simulink model "SEBAS_mario"  (R2013b)
settings: Solver=FixedStepDiscrete  SolverMode=SingleTasking  StartTime=0.0  StopTime=inf  FixedStep=balancer_ts  RelTol=1e-3
undefined symbols (not defined in the file): a_d, a_r, balancerStates_Bus0, Batt, battery_gain, battery_offset, cmd_max, current_mode_status, current_task_operation_status, DiscIntNeverNeededParam, exec_period, Init_Bus0, K, k_f, k_i, k_phidot, k_thetadot, lightCalib, phi_des, R, STATE, TRACK_MODE_LIST, ts2, W
libraries: legonxtlib x29, simulink x19, simulink_extras x4
(part 5 of 5)

== stateflow chart SEBAS_mario/Main Controller/normal_operation_modes.line_tracking_mode ==
  state line_tracking_mode
    entry:
    desired_tail = single(2.0); %radian
    entry, during:
    PWM.tail = tail_controller(sensors.theta_T,desired_tail);
    exit:
    PWM.tail = single(0);
    state Waiting
      entry: debugFlag = uint16(400);
    state Track
      entry:
      BT_status_out = single(StatusID.NXT1_AT_STAGE);
      debugFlag = uint16(401);
      bias = single(0);
      FlagSteering = single(0);
      lineSide = single(1);
      desired_tail = single(0); %radian
      gyroTrick = single(0);
      minLight = lightCalib.flashingWhite;
      maxLight = lightCalib.flashingBlack;
      bias_WhiteSide = lightCalib.flashingWhite + 0.3*(lightCalib.flashingBlack - lightCalib.flashingWhite);
      bias_BlackSide = lightCalib.flashingBlack - 0.45*(lightCalib.flashingBlack - lightCalib.flashingWhite);
      state preProcess [parallel]
        during:
        on every(3, tick):
        [normalizedLight, filteredLight] = processLight(sensors.light, bias, minLight,maxLight);
        [AngleCount,EncoderReset,Angle, Distance] = analyzeEncoders(rawSensors);
        settings: executionOrder=1
      state manageRacePhases [parallel]
        settings: executionOrder=2
        state BeforeShortcut
          entry:
          PID = single([10 0 30 0 90]');
          FlagSteering = single(0);
          bias = single(0);
          state RocketStart1
            state Gyro [parallel]
              settings: executionOrder=1
              state trick
                entry: gyroTrick = single(20);
              state Normal
                entry: gyroTrick = single(0);
              (default) -> trick
              trick -> Normal : after(3*20*0.004,sec)
            state Speed [parallel]
              settings: executionOrder=2
              state slowdown
                entry: fwd = single(130)
                during:
                % fwd = fwd + single(0.005/3);
                fwd = fwd + single(1/2);
              state constantSpeed2
              (default) -> line_tracking_mode.Track.manageRacePhases.BeforeShortcut.RocketStart1.Speed.slowdown
              line_tracking_mode.Track.manageRacePhases.BeforeShortcut.RocketStart1.Speed.slowdown -> line_tracking_mode.Track.manageRacePhases.BeforeShortcut.RocketStart1.Speed.constantSpeed2 : [fwd >= 140]
          state GoUp
            entry:Speak;
            bias = bias_WhiteSide;
            state slowdown
              during:
              fwd = fwd - single(1/2);
            state constantSpeed1
            (default) -> line_tracking_mode.Track.manageRacePhases.BeforeShortcut.GoUp.slowdown
            line_tracking_mode.Track.manageRacePhases.BeforeShortcut.GoUp.slowdown -> line_tracking_mode.Track.manageRacePhases.BeforeShortcut.GoUp.constantSpeed1 : [fwd <= 120]
          state GoDown
            entry:Speak;
            bias = bias_BlackSide;
            state speedup
              during:
              % fwd = fwd + single(1/3)
              fwd = fwd + single(1/4)
            state constantSpeed1
            (default) -> speedup
            speedup -> line_tracking_mode.Track.manageRacePhases.BeforeShortcut.GoDown.constantSpeed1 : [fwd >= 130]
          state Curve
            entry:Speak;
            PID = single([20 0 30 0 100]');
            bias = bias_WhiteSide;
            state slowdown
              during:
              fwd = fwd - single(1/3)
            state constantSpeed2
            (default) -> line_tracking_mode.Track.manageRacePhases.BeforeShortcut.Curve.slowdown
            line_tracking_mode.Track.manageRacePhases.BeforeShortcut.Curve.slowdown -> line_tracking_mode.Track.manageRacePhases.BeforeShortcut.Curve.constantSpeed2 : [fwd <= 120]
          (default) -> RocketStart1
          RocketStart1 -> GoUp : [single(EncoderReset*(2*pi*4.1)/360) >= single(200)]
          GoUp -> GoDown : [single(EncoderReset*(2*pi*4.1)/360) >= single(270)]
          GoDown -> Curve : [single(EncoderReset*(2*pi*4.1)/360) >= single(410)]
        state Shortcut
          state Shortcut
            entry:
            Speak;
            PID = single([18 0 0 0 0]');
            FlagSteering = single(1);
            state slowdown
              during:
              fwd = fwd - single(2)
            state coast
            (default) -> line_tracking_mode.Track.manageRacePhases.Shortcut.Shortcut.slowdown
            line_tracking_mode.Track.manageRacePhases.Shortcut.Shortcut.slowdown -> line_tracking_mode.Track.manageRacePhases.Shortcut.Shortcut.coast : [fwd <= 60]
          state TurnTowardLine
            entry:
            Speak;
            PID = single([0 0 0 0 0]');
            FlagSteering = single(1);
          state skipFirstLine
            entry: Speak;
            EncoderTmp = EncoderReset;
          state SearchLine2
            state TurnLeft
              entry:
              Speak;
              PID = single([25 0 0 0 0]');
              FlagSteering = single(1);
              state slowdown
                during:
                fwd = fwd - single(2)
              state coast
              (default) -> line_tracking_mode.Track.manageRacePhases.Shortcut.SearchLine2.TurnLeft.slowdown
              line_tracking_mode.Track.manageRacePhases.Shortcut.SearchLine2.TurnLeft.slowdown -> line_tracking_mode.Track.manageRacePhases.Shortcut.SearchLine2.TurnLeft.coast : [fwd <= 20]
            state SlowlyApproachLine
              entry:
              Speak;
              fwd = single(20);
              PID = single([-2 0 0 0 0]');
              FlagSteering = single(1);
            (default) -> TurnLeft
            TurnLeft -> SlowlyApproachLine : [Angle >= single(245)]
          state SlowlyRestartLineTracking1
            entry: Speak;
            fwd = single(20);
            PID = single([30 0 25 0 100]');
            bias = single(0);
            FlagSteering = single(0);
          (default) -> line_tracking_mode.Track.manageRacePhases.Shortcut.Shortcut
          line_tracking_mode.Track.manageRacePhases.Shortcut.Shortcut -> TurnTowardLine : [Angle > single(205)]
          TurnTowardLine -> skipFirstLine : [filteredLight>single(0)]
          skipFirstLine -> SearchLine2 : [EncoderReset >= (EncoderTmp + single(200))]
          SearchLine2 -> SlowlyRestartLineTracking1 : %[filteredLight>single(0)]
              | [filteredLight>bias_WhiteSide]
        state AfterShortcut
          state LineFound
            entry:
            debugFlag = uint16(7788);
            Speak;
            %PID = single([30 0 25 0 100]');
            %bias = single(5);
            onMap = false;
            PID = single([20 0 30 0 95]');
            bias = bias_BlackSide;
            FlagSteering = single(0);
            state accelerate
              during:
              % fwd = fwd + single(1/3);
              fwd = fwd + single(1/5);
            state coast
            (default) -> accelerate
            accelerate -> line_tracking_mode.Track.manageRacePhases.AfterShortcut.LineFound.coast : [fwd >= 100]
          state StraightPart
            entry:
            debugFlag = uint16(7789);
            Speak;
            %PID = single([14 0 20 0 70]');
            %bias = single(0);
            PID = single([10 0 30 0 90]');
            bias = bias_WhiteSide;
            FlagSteering = single(0);
            state accelerate1
              during:
              % fwd = fwd + single(1/3);
              fwd = fwd + single(1/2);
            state coast1
            (default) -> line_tracking_mode.Track.manageRacePhases.AfterShortcut.StraightPart.accelerate1
            line_tracking_mode.Track.manageRacePhases.AfterShortcut.StraightPart.accelerate1 -> line_tracking_mode.Track.manageRacePhases.AfterShortcut.StraightPart.coast1 : %[fwd >= 120]
                | [fwd >= 140]
          (default) -> LineFound
          LineFound -> StraightPart : %[Distance >= 10000]
              | [Distance >= 9500]
        state YoshiRide
          state onMap
            entry:
            BT_status_out = single(StatusID.NXT1_AT_STAGE);
            debugFlag = uint16(2201);
            Speak;
            %minLight = single(-95);
            %maxLight = single(32);
            %PID = single([0 0 0 0 0]');
            %bias = single(0);
            %FlagSteering = single(1);
            exit:
            d0 = Distance;
            phi_des = states.phi+single(0*pi/180);
            enablePhiTracking = single(1);
            state accelerate2
              during:
              fwd = fwd - single(1/3);
            state coast2
            (default) -> accelerate2
            accelerate2 -> coast2 : [fwd <= 80]
          state onMap1
            entry:
            debugFlag = uint16(2201);
            Speak;
            minLight = single(-60);
            maxLight = single(90);
            PID = single([30 0 20 0 100]');
            state accelerate1
              during:
              fwd = fwd - single(4/3);
            state coast1
            (default) -> line_tracking_mode.Track.manageRacePhases.YoshiRide.onMap1.accelerate1
            line_tracking_mode.Track.manageRacePhases.YoshiRide.onMap1.accelerate1 -> line_tracking_mode.Track.manageRacePhases.YoshiRide.onMap1.coast1 : [fwd <= 20]
          state GoUp2
            entry:
            Speak;
            phiavg = single(0);
            i = d0+ single(0.75*360);
            PID = single([30 0 20 0 100]');
            bias = single(0);
            FlagSteering = single(0);
            enablePhiTracking = single(1);
            exit:
            phi_des = phiavg/single(6);
            %phi_des = phi_des - single(0.2);
            GoUp2 -> (junction 493) [order 1]
            (junction 493) -> (junction 492) [order 1] : [Distance >= (i+single(0.25*360)) && Distance <= (d0+single(2.3*360))]
            (junction 493) -> (junction 494) [order 2]
            (junction 492) -> (junction 491) : {phiavg = states.phi + phiavg; i = i+single(0.25*360);}
            (junction 491) -> (junction 494)
            (junction 494) -> (junction 490)
          state GoStraightForJump
            entry:
            PID = single([30 0 20 0 100]');
            bias = single(0);
            FlagSteering = single(0);
            enablePhiTracking = single(1);
            minLight = single(-50);
            maxLight = single(65);
          state onMap2
            entry:
            debugFlag = uint16(2201);
            Speak;
            PID = single([0 0 0 0 0]');
            bias = single(0);
            FlagSteering = single(1);
            state accelerate1
              during:
              fwd = fwd - single(4/3);
            state coast1
            (default) -> line_tracking_mode.Track.manageRacePhases.YoshiRide.onMap2.accelerate1
            line_tracking_mode.Track.manageRacePhases.YoshiRide.onMap2.accelerate1 -> line_tracking_mode.Track.manageRacePhases.YoshiRide.onMap2.coast1 : [fwd <= 0]
          state onMap3
            entry:
            enablePhiTracking = single(1);
            debugFlag = uint16(2201);
            Speak;
            PID = single([30 0 25 0 100]');
            bias = single(0);
            FlagSteering = single(0);
            minLight = single(-50);
            maxLight = single(65);
            state accelerate1
              during:
              fwd = fwd + single(1/3);
            state coast1
            (default) -> line_tracking_mode.Track.manageRacePhases.YoshiRide.onMap3.accelerate1
            line_tracking_mode.Track.manageRacePhases.YoshiRide.onMap3.accelerate1 -> line_tracking_mode.Track.manageRacePhases.YoshiRide.onMap3.coast1 : [fwd >= 40]
          state DownRamp
            entry: Speak;
            enablePhiTracking=single(1);
            minLight = single(-5);
            maxLight = single(50);
          state DownRamp1
            entry: Speak;
            enablePhiTracking=single(0);
          (default) -> onMap
          onMap -> onMap1 : [states.balancerStates.theta_dot < single(2.5)]
          onMap1 -> GoUp2 : [Distance >= d0+ single(0.5*360)]
          GoUp2 -> GoStraightForJump [order 1] : [Distance >= d0 + single(2.5*360)]
          GoStraightForJump -> onMap2 : [Distance >= d0 + single(3.4*360)]
          onMap2 -> onMap3 : after(5,sec)
          onMap3 -> DownRamp : [Distance >= d0 +single(3.8.*360)]
          DownRamp -> DownRamp1 : [Distance >= d0 + single(4.5*360)]
        state betweenYoshiAndSeesaw
          state backOnMap
            entry:
            BT_status_out = single(StatusID.NXT1_OFF_RAMP);
            debugFlag = uint16(2201);
            Speak;
            PID = single([30 0 25 0 100]');
            bias = single(0);
            FlagSteering = single(0);
            minLight =lightCalib.flashingMapWhite;
            maxLight = lightCalib.flashingMapBlack;
            enablePhiTracking = single(0);
            state accelerate1
              during:
              fwd = fwd - single(1/3);
            state coast1
            (default) -> line_tracking_mode.Track.manageRacePhases.betweenYoshiAndSeesaw.backOnMap.accelerate1
            line_tracking_mode.Track.manageRacePhases.betweenYoshiAndSeesaw.backOnMap.accelerate1 -> line_tracking_mode.Track.manageRacePhases.betweenYoshiAndSeesaw.backOnMap.coast1 : [fwd <= 20]
          state CrossLine4
            entry:
            Speak;
            PID = single([0 0 0 0 0]');
            bias = single(0);
            FlagSteering = single(1);
          state LineCrossed2
            entry:
            Speak;
            PID = single([30 0 25 0 100]');
            FlagSteering = single(0);
            lineSide = single(-1);
          state backOnMap2
            entry:
            Speak;
            PID = single([30 0 25 0 100]');
            bias = single(0);
            FlagSteering = single(0);
            state accelerate1
              during:
              fwd = fwd + single(1/3);
            state coast1
            (default) -> line_tracking_mode.Track.manageRacePhases.betweenYoshiAndSeesaw.backOnMap2.accelerate1
            line_tracking_mode.Track.manageRacePhases.betweenYoshiAndSeesaw.backOnMap2.accelerate1 -> line_tracking_mode.Track.manageRacePhases.betweenYoshiAndSeesaw.backOnMap2.coast1 : [fwd >= 60]
          state backOnMap4
            entry:
            Speak;
            PID = single([20 0 25 0 100]');
            bias = single(0);
            FlagSteering = single(0);
            state accelerate1
              during:
              fwd = fwd + single(1/3);
            state coast1
            (default) -> line_tracking_mode.Track.manageRacePhases.betweenYoshiAndSeesaw.backOnMap4.accelerate1
            line_tracking_mode.Track.manageRacePhases.betweenYoshiAndSeesaw.backOnMap4.accelerate1 -> line_tracking_mode.Track.manageRacePhases.betweenYoshiAndSeesaw.backOnMap4.coast1 : [fwd >= 120]
          state backOnMap5
            entry:
            Speak;
            PID = single([30 0 25 0 100]');
            bias = single(-10);
            FlagSteering = single(0);
            state accelerate1
              during:
              fwd = fwd - single(1/3);
            state coast1
            (default) -> line_tracking_mode.Track.manageRacePhases.betweenYoshiAndSeesaw.backOnMap5.accelerate1
            line_tracking_mode.Track.manageRacePhases.betweenYoshiAndSeesaw.backOnMap5.accelerate1 -> line_tracking_mode.Track.manageRacePhases.betweenYoshiAndSeesaw.backOnMap5.coast1 : [fwd <= 80]
          (default) -> backOnMap
          backOnMap -> CrossLine4 : [Distance >= d0 + single(7.2*360)]
          CrossLine4 -> LineCrossed2 : after(0.2,sec)
          LineCrossed2 -> backOnMap2 : after(1,sec)
          backOnMap2 -> backOnMap4 : [Distance >= d0 + single(10.5*360)]
          backOnMap4 -> backOnMap5 : [Distance >= d0 + single(12.5*360)]{Speak}
        state Jump
          entry:
          Speak;
          phiavg = single(0);
          i = d0+ single(17*360);
          PID = single([30 0 20 0 100]');
          bias = single(0);
          FlagSteering = single(0);
          enablePhiTracking = single(0);
          exit:
          phi_des = phiavg/single(7);
          Jump -> (junction 515) [order 1]
          (junction 515) -> (junction 509) [order 1] : [Distance >= (i+single(0.2*360)) && Distance <= (d0+single(1.5*360))]
          (junction 515) -> (junction 516) [order 2]
          (junction 509) -> (junction 519) : {phiavg = states.phi + phiavg; i = i+single(0.2*360);}
          (junction 519) -> (junction 516)
          (junction 516) -> (junction 520)
        state Done
          entry:
          Speak;
          turnLightOn;
          PWM.left = single(0); PWM.right = single(0);
          current_mode_status = OperationModeStatusEnum.SUCCESSFULLY_COMPLETED;
        (default) -> BeforeShortcut
        StraightPart -> YoshiRide : [Distance >= 12000]
        Jump -> Done [order 1] : [Distance >= d0 + single(18.5*360)]{Speak;}
        Curve -> line_tracking_mode.Track.manageRacePhases.Shortcut : [Distance >= single(7200)]
        DownRamp1 -> betweenYoshiAndSeesaw : [Distance >= d0 + single(6*360)]
        SlowlyRestartLineTracking1 -> AfterShortcut : after(1,sec)
        backOnMap5 -> Jump : [Distance >= d0 + single(17*360)]{Speak;}
      state ApplyControl [parallel]
        during:
        on every(3, tick):  lineTrackCmd = lineTracker(normalizedLight,FlagSteering,PID,fwd)
        during:
        %lineTrackCmd(2) = lineSide*lineTrackCmd(2);
        if lineSide >0
        [PWM.left PWM.right] = balanceControl(rawSensors,lineTrackCmd,gyroTrick);
        if enablePhiTracking
        PWM.left = PWM.left + phiController(states.phi,phi_des,sensors.battery);
        PWM.right = PWM.right - phiController(states.phi,phi_des,sensors.battery);
        end
        else
        [PWM.right PWM.left] = balanceControl(rawSensors,lineTrackCmd,gyroTrick);
        if enablePhiTracking
        PWM.left = PWM.left - phiController(states.phi,phi_des,sensors.battery);
        PWM.right = PWM.right + phiController(states.phi,phi_des,sensors.battery);
        end
        end
        settings: executionOrder=3
      state [normalizedLight,filteredLight] = processLight(rawLight,bias,minLight,maxLight) [function]
      state [AngleCount,EncoderReset,Angle,Distance] = analyzeEncoders(rawSensors) [function]
      state cmd = lineTracker(lightSignal,flagSteering,PID,fwd) [function]
    state cmd = phiController(phi,desiredPhi,battery) [function]
    state [leftPWM,rightPWM] = balanceControl(rawSensors,lineTrackCmd,gyroTrick) [function]
    state cmd = tail_controller(current,desired) [function]
    state turnLightOn [function]
    state Speak [function]
    (default) -> Waiting
    Waiting -> Track : [hasChangedFrom(touch,single(0))]
  data: rawLight function_input single size=1; bias function_input single size=1; normalizedLight function_output single size=1; filteredLight function_output single size=1; minLight function_input single size=1; maxLight function_input single size=1; rawSensors function_input Bus: Sensors_Bus size=1; AngleCount function_output uint8 size=1; EncoderReset function_output single size=1; Angle function_output single size=1; Distance function_output single size=1; lightSignal function_input single size=1; flagSteering function_input single size=1; PID function_input single size=5; fwd function_input single size=1; cmd function_output; cmd function_output; phi function_input single size=1; desiredPhi function_input single size=1; battery function_input double size=1; leftPWM function_output single size=1; rawSensors function_input Bus: Sensors_Bus size=1; rightPWM function_output; lineTrackCmd function_input single size=2; gyroTrick function_input single size=1; current function_input single size=1; desired function_input single size=1; cmd function_output single size=1; sensors input Bus: Sensors_Bus size=1; touch input single size=1; PWM output Bus: PWM_bus size=1; debugFlag output uint16 size=1; current_mode_status data_store_memory; desired_tail local single size=1; states input Bus: States_Bus size=1; rawSensors input Bus: Sensors_Bus size=1; lineTrackCmd local single size=2; PID local single size=5; normalizedLight local single size=1; AngleCount local uint8 size=1; EncoderReset local single size=1; Angle local single size=1; bias local single size=1; fwd local single size=1; FlagSteering local single size=1; filteredLight local single; EncoderTmp local single size=1; Distance local single size=1; phi_des data_store_memory size=1; enablePhiTracking local; d0 local; lineSide local; phiavg local single size=1; i local single size=1; lightCalib data_store_memory; gyroTrick local; bias_WhiteSide local; bias_BlackSide local; minLight local single size=1; maxLight local single size=1; onMap local; BT_status_out output single

== stateflow chart SEBAS_mario/Main Controller/normal_operation_modes.light_calibration_up ==
  state wait
    entry:debugFlag = uint16(200);
  state MoveUp
    entry:debugFlag = uint16(201);
    PWM.tail = single(-50);
  state Reset
    entry:debugFlag = uint16(202);
    PWM.tail = single(0);
    initFlags.tail = single(1);
    exit:
    initFlags.tail = single(0);
    desired_tail = single(0);
  state light_sensor_calibration_up
    %during, exit: PWM.tail = tail_controller(sensors.theta_T,single(1.6))
    state WaitForBlack
      entry: debugFlag = uint16(310);
    state StoreBlack
      entry: lightCalib.black = sensors.light;
      debugFlag = uint16(311);
    state WaitForWhite
      entry: debugFlag = uint16(312)
    state StoreWhite
      entry: lightCalib.white = sensors.light;
      debugFlag = uint16(313);
    state CalibComplete
      entry:
      debugFlag = uint16(318);
      current_task_operation_status = OperationModeStatusEnum.SUCCESSFULLY_COMPLETED;
    state cmd = tail_controller(current,desired) [function]
    (default) -> WaitForBlack
    WaitForBlack -> StoreBlack : [hasChangedFrom(touch,single(0))]
    StoreBlack -> WaitForWhite : after(0.2,sec){Speak;}
    WaitForWhite -> StoreWhite : [hasChangedFrom(touch,single(0))]
    StoreWhite -> CalibComplete : after(0.2,sec){Speak;}
  state Speak [function]
  (default) -> wait
  wait -> MoveUp : [hasChangedFrom(touch,single(0))]{Speak;}
  MoveUp -> Reset : after(2,sec)
  Reset -> light_sensor_calibration_up : after(1,sec){Speak;}
  data: current function_input single size=1; desired function_input single size=1; cmd function_output single size=1; sensors input Bus: Sensors_Bus size=1; lightCalib data_store_memory; current_task_operation_status data_store_memory; debugFlag output uint16; touch input single size=1; PWM output Bus: PWM_bus size=1; initFlags output Bus: Init_Bus size=1; desired_tail local

== stateflow chart SEBAS_mario/Main Controller/normal_operation_modes.light_calibration_up_flashing_on_map ==
  state LightSensorCalibFlashing
    during:
    on every(3, tick): filteredLight = processLight(sensors.light);
    state WaitForBlack
      entry: debugFlag = uint16(310);
    state StoreBlack
      entry: lightCalib.flashingMapBlack = filteredLight;
      debugFlag = uint16(311);
      Speak;
    state WaitForWhite
      entry: debugFlag = uint16(312);
      Speak;
    state StoreWhite
      entry: lightCalib.flashingMapWhite = filteredLight;
      debugFlag = uint16(313);
      Speak;
      exit:
      turnLightOn;
      Speak;
    state CalibComplete
      entry:
      debugFlag = uint16(318);
      current_task_operation_status = OperationModeStatusEnum.SUCCESSFULLY_COMPLETED;
    state cmd = tail_controller(current,desired) [function]
    state Speak [function]
    state turnLightOn [function]
    state filteredLight  = processLight(rawLight) [function]
    (default) -> WaitForBlack
    WaitForBlack -> StoreBlack : [hasChangedFrom(touch,single(0))]
    StoreBlack -> WaitForWhite : after(1,sec)
    WaitForWhite -> StoreWhite : [hasChangedFrom(touch,single(0))]
    StoreWhite -> CalibComplete : after(1,sec)
  data: current function_input single size=1; desired function_input single size=1; cmd function_output single size=1; rawLight function_input single size=1; filteredLight function_output single size=1; sensors input Bus: Sensors_Bus size=1; lightCalib data_store_memory; current_task_operation_status data_store_memory; debugFlag output uint16; touch input single size=1; filteredLight local
